simulink model "Simulation_H_bridge"  (R2020b)
settings: Solver=ode23tb  StartTime=0.0  StopTime=stop_time  MaxStep=max_step_size  RelTol=tolerance  EnableMultiTasking=on
values from neighbouring files (symbols this model uses):
  E_ch = -140    [init_cstes_IGBT.m]
  f_sw = 2e3    (= 2000)    [init_cstes.m]    (also in init_cstes_IGBT.m; init_cstes_filter.m)
  L_ch = 10e-3    (= 0.01)    [init_cstes_IGBT.m]
  R_ch = 0.2    [init_cstes_IGBT.m]
  R_i = 1e-6    (= 1e-06)    [init_cstes.m]    (also in init_cstes_IGBT.m; init_cstes_filter.m)
  V_AB_ref = E_ch + R_ch * I_ref    (= -150)    [init_cstes_IGBT.m]
  V_b = 200    [init_cstes.m]    (also in init_cstes_IGBT.m; init_cstes_filter.m)
libraries: powerlib x10, powerlib_meascontrol x4, simulink x1
settings Model: Creator=ULB  LastModifiedBy=arnaudsaison
settings SolverCC: SolverResetMethod=Robust
settings DataIOCC: LimitDataPoints=on  SaveFormat=Array  SignalLoggingSaveFormat=ModelDataLogs  ReturnWorkspaceOutputs=off
settings OptimizationCC: ExpressionDepthLimit=2147483647  LifeSpan=inf
settings DebuggingCC: UnderspecifiedInitializationDetection=Classic  MergeDetectMultiDrivingBlocksExec=none  SolverPrmCheckMsg=warning  FcnCallInpInsideContextMsg=warning  UnconnectedInputMsg=none  UnconnectedOutputMsg=none  UnconnectedLineMsg=none  StateNameClashWarn=warning  SFUnexpectedBacktrackingDiag=warning  SFNoUnconditionalDefaultTransitionDiag=warning  SFExecutionAtInitializationDiag=none  ArithmeticOperatorsInVariantConditions=warning
settings HardwareCC: ProdBitPerPointer=32  ProdBitPerSizeT=32  ProdBitPerPtrDiffT=32  ProdLargestAtomicFloat=None  ProdIntDivRoundTo=Undefined  ProdEndianess=Unspecified  ProdWordSize=32  ProdHWDeviceType=32-bit Generic
settings ModelReferenceCC: PropagateSignalLabelsOutOfModel=off
settings SFSimCC: SimUseLocalCustomCode=off  CustomCodeUndefinedFunction=UseInterfaceOnly
settings RTWCC: RTWUseLocalCustomCode=off
settings CodeAppCC: StateflowObjectComments=on
settings GRTTargetCC: TargetLangStandard=C89/C90 (ANSI)  CombineOutputUpdateFcns=off  GRTInterface=on
settings ConfigComp: CovMetricSettings=dw  CovSaveCumulativeToWorkspaceVar=on  CovSaveSingleToWorkspaceVar=on  CovExternalEMLEnable=off
settings SimscapeCC: SimscapeNormalizeSystem=off

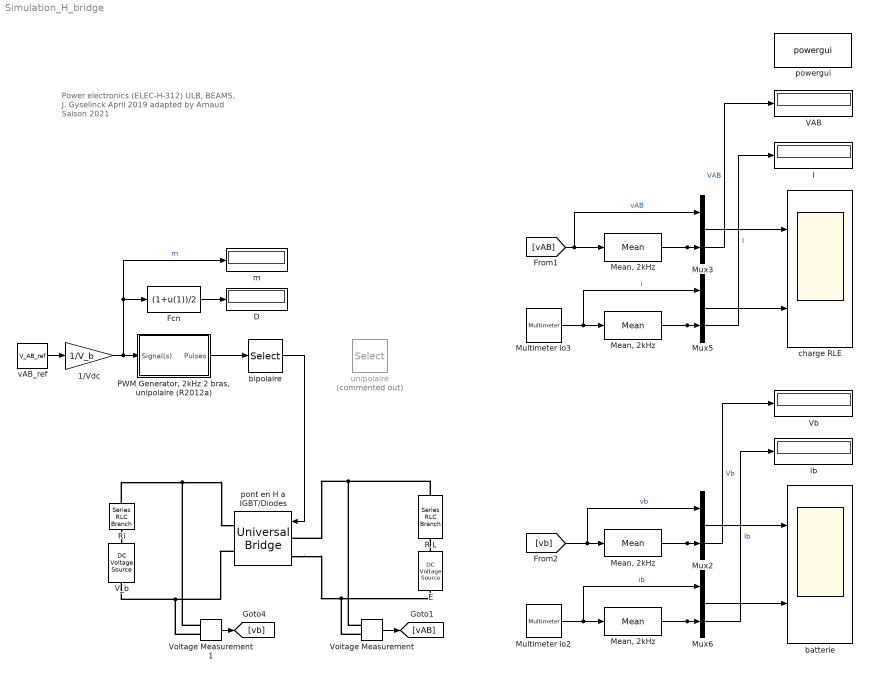
== system Simulation_H_bridge ==
  note: Power electronics (ELEC-H-312)
      | ULB, BEAMS, J. Gyselinck April 2019
      | adapted by Arnaud Saison 2021
  "   Mean, 2kHz   " : powerlib_meascontrol/Measurements/Mean  Freq=f_sw  Vinit=0  Ts=0
  "  Mean, 2kHz " : powerlib_meascontrol/Measurements/Mean  Freq=f_sw  Vinit=0  Ts=0
  "  Mean, 2kHz  " : powerlib_meascontrol/Measurements/Mean  Freq=f_sw  Vinit=0  Ts=0
  1/Vdc : Gain  Gain=1/V_b
  D : Display
      settings: Format=short_e
  E : powerlib/Electrical Sources/DC Voltage Source  Amplitude=E_ch  Measurements=None
  Fcn : Fcn  Expr=(1+u(1))/2
  I : Display
      settings: Format=short_e
  Ib : Display
      settings: Format=short_e
  "Mean, 2kHz" : powerlib_meascontrol/Measurements/Mean  Freq=f_sw  Vinit=0  Ts=0
  Multimeter io2 : powerlib/Measurements/Multimeter  PhasorSimulation=off  OutputType=Complex  sel=10  L=14  Gain=1  yselected={'Ib: Ri'};  PSBOutputType=1  PSBequivalent=0  AxesSetting=[0,0.1,-100,100]  Display=0  SavedBlockNames=-11
  Multimeter io3 : powerlib/Measurements/Multimeter  PhasorSimulation=off  OutputType=Complex  sel=9  L=14  Gain=1  yselected={'Ib: R L'};  PSBOutputType=1  PSBequivalent=0  AxesSetting=[0,0.1,-100,100]  Display=0  SavedBlockNames=-11
  Mux{2..3,5..6} (4 alike) : Mux  Inputs=2
  "PWM Generator, 2kHz 2 bras, unipolaire (R2012a)" : Subsystem  AncestorBlock="powerlib_extras/Control  Blocks/PWM Generator"  DialogController=POWERSYS.PowerSysDialog  mask(PWM Generator){GeneratorMode=2-arm  bridge (4 pulses), Fc=f_sw, Internal=off, mIndex=0.4, Freq=60, Phase=0}
      mask prompts: GeneratorMode "Generator Mode"; Fc "Carrier frequency (Hz):"; Internal "Internal generation of modulating signal(s)"; mIndex "Modulation index  (0<m<1) :"; Freq "Frequency of output voltage (Hz)"; Phase "Phase of output voltage (degrees)"
      mask help:
      | This block generates pulses for carrier-based PWM (Pulse Width Modulation), self-commutated IGBTs,GTOs or FETs bridges.
      |
      | Depending on the number of bridge arms selected in the "Generator Mode" parameter, the block can be used either for single-phase or three-phase PWM control.
      mask init:
      | if Freq==0
      |     Phase=90;
      | end
      | switch GeneratorMode
      | case 1,
      |     Internal_Phase=0;
      |    Signal_PortWidth=1;
      |    Select1_Elements=[1 2];
      |    Select1_PortWidth=2;
      |    Select3_Elements=[1 2];
      |    Select3_PortWidth=4;
      | case 2,
      |     Internal_Phase=0;
      |     Signal_PortWidth=1;
      |     Select1_Elements=[1 2];
      |     Select1_PortWidth=2;
      |     Select3_Elements=[1 2 3 4];
      |     Select3_PortWidth=4;
      | case 3,
      |     Internal_Phase=[0 -2*pi/3 2*pi/3];
      |     Signal_PortWidth=3;
      |     Select1_Elements=[1 4 2 5 3 6];
      |     Select1_PortWidth=6;
      |    Select3_Elements=[1 2 3 4 5 6];
      |    Select3_PortWidth=12;
      | case 4,
      |     Internal_Phase=[0 -2*pi/3 2*pi/3];
      |     Signal_PortWidth=3;
      |     Select1_Elements=[1 4 2 5 3 6];
      |     Select1_PortWidth=6;
      |    Select3_Elements=[1 2 3 4 5 6 7 8 9 10 11 12];
      |    Select3_PortWidth=12;
      | end
      | power_initmask();
      mask Help: web(psbhelp)
      mask TypeOptions GeneratorMode: 1-arm  bridge (2 pulses) | 2-arm  bridge (4 pulses) | 3-arm  bridge (6 pulses) | Double 3-arm  bridges (12 pulses)
      mask Callback Internal: p3=get_param(gcb,'Internal');if strcmp(p3,'on');visible={'on','on','on','on','on','on'};else;visible={'on','on','on','off','off','off'};end;set_param(gcb,'MaskVisibilities',visible)
  R L : powerlib/Elements/Series RLC Branch  LConnTagsString=__new0  RConnTagsString=__new0  BranchType=RL  Resistance=R_ch  Inductance=L_ch  SetiL0=off  InitialCurrent=0  Capacitance=1e-6  Setx0=off  InitialVoltage=0  Measurements=Branch voltage and current
  Ri : powerlib/Elements/Series RLC Branch  LConnTagsString=__new0  RConnTagsString=__new0  BranchType=R  Resistance=R_i  Inductance=2e-3  SetiL0=off  InitialCurrent=0  Capacitance=1e-6  Setx0=off  InitialVoltage=0  Measurements=Branch voltage and current
  VAB : Display
      settings: Format=short_e
  V_b : powerlib/Electrical Sources/DC Voltage Source  Amplitude=V_b  Measurements=None
  Vb : Display
      settings: Format=short_e
  Voltage Measurement : powerlib/Measurements/Voltage Measurement  PhasorSimulation=off  OutputType=Complex  PSBequivalent=0
  Voltage Measurement1 : powerlib/Measurements/Voltage Measurement  PhasorSimulation=off  OutputType=Complex  PSBequivalent=0
  batterie : Scope  NumInputPorts=2
  bipolaire : Selector  InputPortWidth=4  IndexOptions=Index vector (dialog)  Indices=[1 2 2 1]  OutputSizes=1
  charge RLE : Scope  NumInputPorts=2
  m : Display
      settings: Format=short_e
  pont en H a IGBT/Diodes : powerlib/Power Electronics/Universal Bridge  Arms=2  SnubberResistance=999  SnubberCapacitance=999  Device=IGBT / Diodes  Ron=999  Lon=0  ForwardVoltages=[ 999 , 999 ]  ForwardVoltage=0  GTOparameters=[ 10e-6 , 20e-6 ]  IGBTparameters=[ 333 , 333 ]  Measurements=All voltages and currents  Measurements_2=None  converterType=Rectifier
  powergui : powerlib/powergui  SimulationMode=Continuous  SampleTime=1e-6  frequency=60  Iterations=50  frequencyindice=0  Pbase=100e6  ErrMax=1e-4  UnitsV=kV  UnitsW=MW  buscounter=0  FunctionMessages=off  echomessages=off  EnableUseOfTLC=off  CurrentSourceSwitches=off  DisableSnubberDevices=off  DisableRonSwitches=on  DisableVfSwitches=on  DisplayEquations=off  AutomaticDiscreteSolvers=off  SolverType=Tustin  Interpol=off  ExternalGateDelay=off  methode=off  Ts=0  x0status=blocks  SPID=off  SwTol=0  HookPort=off  NonlinearTolerance=1e-4  nMaxIteration=100  ContinueOnMaxIteration=off  RestoreLinks=warning  ResistiveCurrentMeasurement=off  Frange=[0:2:500]  Ylog=off  Xlog=on  ShowGrid=off  save=off  variable=ZData  structure=vio  ZoomFFT=off  StartTime=0.1  cycles=3  DisplayStyle=4  fundamental=50  FreqAxis=off  MaxFrequency=3000  frequencyindicesteady=1  RmsSteady=1  display=off
  unipolaire : Selector  Commented=on  InputPortWidth=4  IndexOptions=Index vector (dialog)  Indices=[1 2 3 4]  OutputSizes=1
  vAB_ref : Constant  Value=V_AB_ref
  wires:
  Voltage Measurement/1 -> [vAB]
  vAB_ref/1 -> 1/Vdc/1
  bipolaire/1 -> pont en H a IGBT/Diodes/1
  Voltage Measurement1/1 -> [vb]
  1/Vdc/1 -> m/1, Fcn/1, "PWM Generator, 2kHz 2 bras, unipolaire (R2012a)"/1(Signal(s))  "m"
  "PWM Generator, 2kHz 2 bras, unipolaire (R2012a)"/1(Pulses) -> bipolaire/1
  Fcn/1 -> D/1
  Mux5/1 -> charge RLE/2
  Mux3/1 -> charge RLE/1
  Multimeter io3/1 -> "Mean, 2kHz"/1, Mux5/1  "i"
  "   Mean, 2kHz   "/1 -> Mux6/2, Ib/1  "Ib"
  Multimeter io2/1 -> "   Mean, 2kHz   "/1, Mux6/1  "ib"
  [vb] -> Mux2/1, "  Mean, 2kHz  "/1  "vb"
  Mux2/1 -> batterie/1
  [vAB] -> Mux3/1, "  Mean, 2kHz "/1  "vAB"
  "  Mean, 2kHz "/1 -> VAB/1, Mux3/2  "VAB"
  "Mean, 2kHz"/1 -> I/1, Mux5/2  "I"
  "  Mean, 2kHz  "/1 -> Vb/1, Mux2/2  "Vb"
  Mux6/1 -> batterie/2
  connections:
  pont en H a IGBT/Diodes/RConn2 -- Voltage Measurement1/LConn2 -- V_b/LConn1
  R L/LConn1 -- Voltage Measurement/LConn1 -- pont en H a IGBT/Diodes/LConn1
  pont en H a IGBT/Diodes/LConn2 -- Voltage Measurement/LConn2 -- E/LConn1
  E/RConn1 -- R L/RConn1
  Ri/RConn1 -- Voltage Measurement1/LConn1 -- pont en H a IGBT/Diodes/RConn1
  Ri/LConn1 -- V_b/RConn1

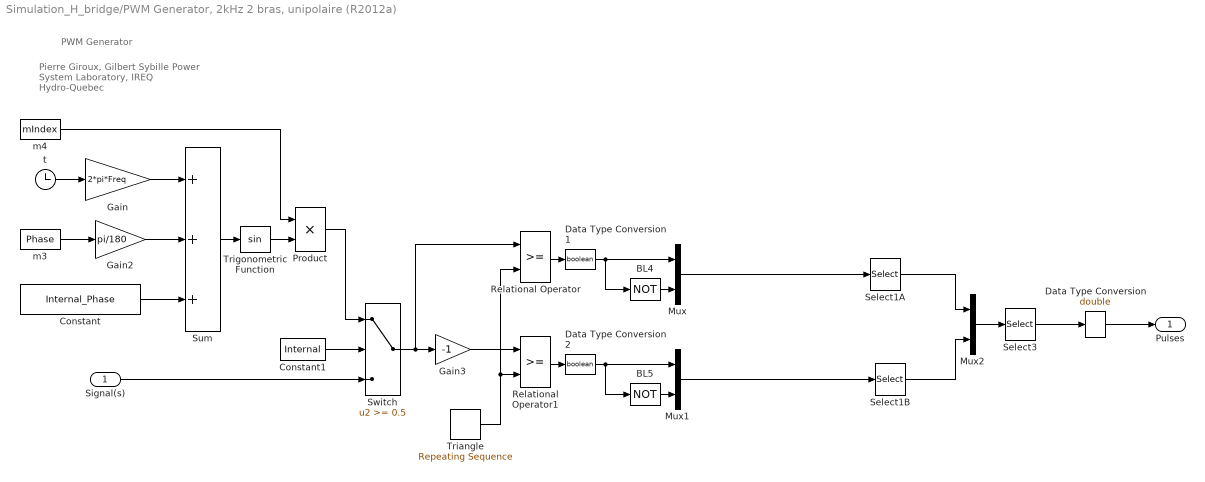
== system Simulation_H_bridge/PWM Generator, 2kHz 2 bras, unipolaire (R2012a) ==
  note: Pierre Giroux, Gilbert Sybille
      | Power System Laboratory, IREQ
      | Hydro-Quebec
  note: PWM Generator
  Signal(s) : Inport  PortDimensions=Signal_PortWidth
  BL4 : Logic  Operator=NOT  Inputs=1
  BL5 : Logic  Operator=NOT  Inputs=1
  Constant : Constant  Value=Internal_Phase
  Constant1 : Constant  Value=Internal
  Data Type Conversion : DataTypeConversion  OutDataTypeStr=double  SaturateOnIntegerOverflow=on  RndMeth=Zero
  Data Type Conversion1 : DataTypeConversion  OutDataTypeStr=boolean  SaturateOnIntegerOverflow=on  RndMeth=Zero
  Data Type Conversion2 : DataTypeConversion  OutDataTypeStr=boolean  SaturateOnIntegerOverflow=on  RndMeth=Zero
  Gain : Gain  Gain=2*pi*Freq  SaturateOnIntegerOverflow=on  OutDataTypeStr=Inherit: Same as input  ParamDataTypeStr=Inherit: Same as input
  Gain2 : Gain  Gain=pi/180  SaturateOnIntegerOverflow=on  OutDataTypeStr=Inherit: Same as input  ParamDataTypeStr=Inherit: Same as input
  Gain3 : Gain  Gain=-1  SaturateOnIntegerOverflow=on  OutDataTypeStr=Inherit: Same as input  ParamDataTypeStr=Inherit: Same as input
  Mux : Mux  Inputs=2
  Mux1 : Mux  Inputs=2
  Mux2 : Mux  Inputs=2
  Product : Product  InputSameDT=on  SaturateOnIntegerOverflow=on  OutDataTypeStr=Inherit: Same as first input
  Relational Operator : RelationalOperator  RndMeth=Nearest  InputSameDT=on
  Relational Operator1 : RelationalOperator  RndMeth=Nearest  InputSameDT=on
  Select1A : Selector  InputPortWidth=Select1_PortWidth  IndexOptions=Index vector (dialog)  Indices=Select1_Elements  OutputSizes=1
  Select1B : Selector  InputPortWidth=Select1_PortWidth  IndexOptions=Index vector (dialog)  Indices=Select1_Elements  OutputSizes=1
  Select3 : Selector  InputPortWidth=Select3_PortWidth  IndexOptions=Index vector (dialog)  Indices=[1 2 3 4]  OutputSizes=1
  Sum : Sum  Inputs=+++  InputSameDT=on  SaturateOnIntegerOverflow=on  OutDataTypeStr=Inherit: Same as first input
  Switch : Switch  Threshold=0.5  InputSameDT=on
  Triangle : simulink/Sources/Repeating Sequence  rep_seq_t=[0 1/Fc/4 3/Fc/4 1/Fc]  rep_seq_y=[0 -1 1 0]
  Trigonometric Function : Trigonometry
  m3 : Constant  Value=Phase
  m4 : Constant  Value=mIndex
  t : Clock
  Pulses : Outport  VectorParamsAs1DForOutWhenUnconnected=off
  wires:
  Triangle/1 -> Relational Operator/2, Relational Operator1/2
  Switch/1 -> Relational Operator/1, Gain3/1
  Mux2/1 -> Select3/1
  Select1B/1 -> Mux2/2
  Select1A/1 -> Mux2/1
  Mux1/1 -> Select1B/1
  Mux/1 -> Select1A/1
  BL5/1 -> Mux1/2
  BL4/1 -> Mux/2
  Gain3/1 -> Relational Operator1/1
  Product/1 -> Switch/1
  Constant1/1 -> Switch/2
  Signal(s)/1 -> Switch/3
  Trigonometric Function/1 -> Product/2
  Sum/1 -> Trigonometric Function/1
  m4/1 -> Product/1
  Constant/1 -> Sum/3
  m3/1 -> Gain2/1
  Gain2/1 -> Sum/2
  Gain/1 -> Sum/1
  t/1 -> Gain/1
  Select3/1 -> Data Type Conversion/1
  Data Type Conversion/1 -> Pulses/1
  Relational Operator/1 -> Data Type Conversion1/1
  Data Type Conversion1/1 -> BL4/1, Mux/1
  Relational Operator1/1 -> Data Type Conversion2/1
  Data Type Conversion2/1 -> BL5/1, Mux1/1
